simulink model "Problem_4_Realize_The_Filter"  (R2020b)
settings: Solver=VariableStepAuto  StartTime=0.0  StopTime=10.0  RelTol=1e-3
libraries: simulink x1
settings Model: Creator=Manoj  LastModifiedBy=Windows 10

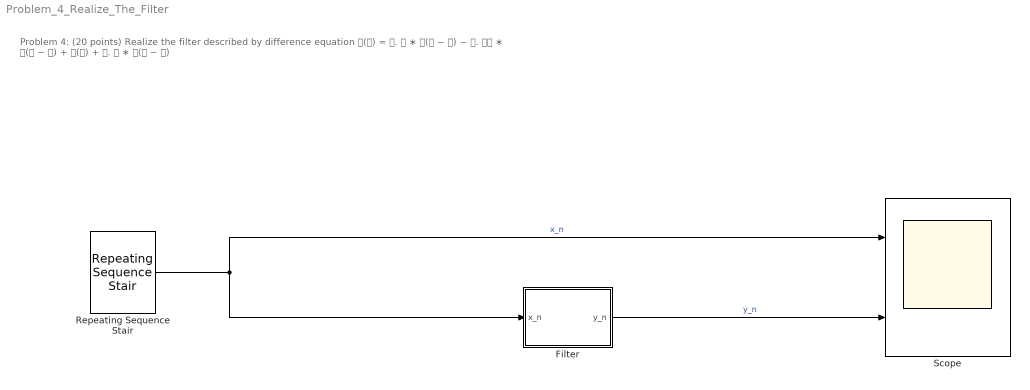
== system Problem_4_Realize_The_Filter ==
  note: Problem 4: (20 points) Realize the filter described by difference equation
      | 𝐲(𝐧) = 𝟎. 𝟓 ∗ 𝐲(𝐧 − 𝟏) − 𝟎. 𝟐𝟓 ∗ 𝐲(𝐧 − 𝟐) + 𝐱(𝐧) + 𝟎. 𝟒 ∗ 𝐱(𝐧 − 𝟏)
  Filter : Subsystem
  Repeating Sequence Stair : simulink/Sources/Repeating Sequence Stair  OutValues=[1 0 0 0 1 0 0 0].'  tsamp=-1  OutMin=[]  OutMax=[]  OutDataTypeStr=double  OutputDataTypeScalingMode=double  OutDataType=fixdt(0,8)  ConRadixGroup=Best Precision: Vector-wise  OutScaling=2^-12
  Scope : Scope  NumInputPorts=2
  wires:
  Repeating Sequence Stair/1 -> Filter/1(x_n), Scope/1  "x_n"
  Filter/1(y_n) -> Scope/2  "y_n"

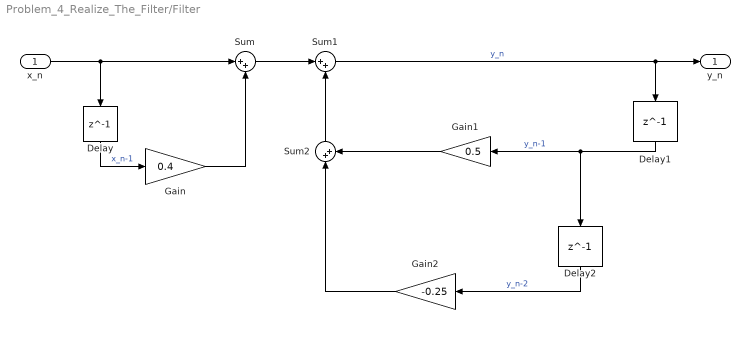
== system Problem_4_Realize_The_Filter/Filter ==
  x_n : Inport
  Delay : Delay  DelayLength=1
  Delay1 : Delay  DelayLength=1
  Delay2 : Delay  DelayLength=1
  Gain : Gain  Gain=0.4
  Gain1 : Gain  Gain=0.5
  Gain2 : Gain  Gain=-0.25
  Sum : Sum  Inputs=|++
  Sum1 : Sum  Inputs=|++
  Sum2 : Sum  Inputs=|++
  y_n : Outport
  wires:
  Gain/1 -> Sum/2
  Delay/1 -> Gain/1  "x_n-1"
  Gain2/1 -> Sum2/1
  x_n/1 -> Sum/1, Delay/1
  Sum2/1 -> Sum1/2
  Delay2/1 -> Gain2/1  "y_n-2"
  Sum1/1 -> y_n/1, Delay1/1  "y_n"
  Delay1/1 -> Gain1/1, Delay2/1  "y_n-1"
  Gain1/1 -> Sum2/2
  Sum/1 -> Sum1/1
